simulink model "ofdmexample1"  (R2017a)
settings: Solver=FixedStepDiscrete  StartTime=0.0  StopTime=0.1  RelTol=1e-3
PostLoadFcn:
  | prm80216d.blkh = []; prm80216d.action = 'init';
  | commwman80216d_init(prm80216d.blkh, prm80216d.action);
  | if isempty(ans), clear ans; end
StartFcn:
  | if isempty(ans), clear ans; end
undefined symbols (not defined in the file): idx, magnitude
libraries: commwman80216d_lib x49, dspsigops x24, commcnvcod2 x14, dspindex x4, commdigbbndpm3 x3, dspsolvers x2, simulink x2, commrflib2 x2, commofdm x2, commsink2 x1, commblksprivate x1, dspmtrx3 x1
(part 2 of 2)

== system ofdmexample1/FEC & Modulator Bank/RateID5 - 64 QAM 2//3 ==
  In1 : Inport
  Enable : EnablePort  PropagateVarSize=During execution
  64-QAM Modulator5 : commwman80216d_lib/64-QAM Modulator  SystemSampleTime=-1
      settings: SourceProductName=Communications System Toolbox  SourceProductBaseCode=CM
  Interleaver5 : commwman80216d_lib/Interleaver  numSubCh=16  Ncbps1=1152  Ncbps2=96  Ncbps3=48  Ncbps4=96  Ncbps5=12  Ncpc=6  numSym=prm80216d.numOFDMSymbols
      settings: SourceProductName=Communications System Toolbox  SourceProductBaseCode=CM
  Punctured Convolutional Encoder5 : commcnvcod2/Convolutional Encoder  trellis=poly2trellis(7, [171 133])  opMode=Truncated (reset every frame)  DelayedResetAction=off  hasIniStPort=off  hasFinStPort=off  usePuncVector=on  punctureVector=reshape([1 0 1;1 1 0 ],6,1)  reset=Unused parameter value
      settings: SourceProductName=Communications System Toolbox  SourceProductBaseCode=CM
  RS Encoder5 : commwman80216d_lib/RS Encoder  N=108  K=96  numSym=prm80216d.numOFDMSymbols
      settings: SourceProductName=Communications System Toolbox  SourceProductBaseCode=CM
  Select Bits : dspsigops/Pad  padAlong=Columns  dimsToPad=1  valSrc=Specify via dialog  padVal=0  spec=Output size  padNumOutRowsSpecMethod=User-specified  numOutRows=prm80216d.uncBlkSize(6)*8*prm80216d.numOFDMSymbols - 8  padNumOutColsSpecMethod=User-specified  numOutCols=1  isVarDimsMode=off  padBeginning=0  padEnd=0  outSizeMode=User-specified  outSize=1  padSigAt=End  trunc_flag=None  roundingMode=Floor  overflowMode=off  truncOrWrapMode=Truncate  wrap_flag=None
      settings: AttributesFormatString=\n  SourceProductName=DSP System Toolbox  SourceProductBaseCode=DS
  Zero pad tail byte : dspsigops/Pad  padAlong=Columns  dimsToPad=1  valSrc=Specify via dialog  padVal=0  spec=Output size  padNumOutRowsSpecMethod=User-specified  numOutRows=prm80216d.uncBlkSize(6)*8*prm80216d.numOFDMSymbols  padNumOutColsSpecMethod=User-specified  numOutCols=1  isVarDimsMode=off  padBeginning=0  padEnd=0  outSizeMode=User-specified  outSize=1  padSigAt=End  trunc_flag=None  roundingMode=Floor  overflowMode=off  truncOrWrapMode=Truncate  wrap_flag=None
      settings: AttributesFormatString=\n  SourceProductName=DSP System Toolbox  SourceProductBaseCode=DS
  Out1 : Outport
  wires:
  RS Encoder5/1 -> Punctured Convolutional Encoder5/1
  Punctured Convolutional Encoder5/1 -> Interleaver5/1
  Interleaver5/1 -> 64-QAM Modulator5/1
  In1/1 -> Select Bits/1
  64-QAM Modulator5/1 -> Out1/1
  Select Bits/1 -> Zero pad tail byte/1
  Zero pad tail byte/1 -> RS Encoder5/1

== system ofdmexample1/FEC & Modulator Bank/RateID6 - 64QAM 3//4 ==
  In1 : Inport
  Enable : EnablePort  PropagateVarSize=During execution
  64-QAM Modulator6 : commwman80216d_lib/64-QAM Modulator  SystemSampleTime=-1
      settings: SourceProductName=Communications System Toolbox  SourceProductBaseCode=CM
  Interleaver6 : commwman80216d_lib/Interleaver  numSubCh=16  Ncbps1=1152  Ncbps2=96  Ncbps3=48  Ncbps4=96  Ncbps5=12  Ncpc=6  numSym=prm80216d.numOFDMSymbols
      settings: SourceProductName=Communications System Toolbox  SourceProductBaseCode=CM
  Punctured Convolutional Encoder6 : commcnvcod2/Convolutional Encoder  trellis=poly2trellis(7, [171 133])  opMode=Truncated (reset every frame)  DelayedResetAction=off  hasIniStPort=off  hasFinStPort=off  usePuncVector=on  punctureVector=reshape([1 0 1 0 1;1 1 0 1 0], 10, 1)  reset=Unused parameter value
      settings: SourceProductName=Communications System Toolbox  SourceProductBaseCode=CM
  RS Encoder6 : commwman80216d_lib/RS Encoder  N=120  K=108  numSym=prm80216d.numOFDMSymbols
      settings: SourceProductName=Communications System Toolbox  SourceProductBaseCode=CM
  Select Bits : dspsigops/Pad  padAlong=Columns  dimsToPad=1  valSrc=Specify via dialog  padVal=0  spec=Output size  padNumOutRowsSpecMethod=User-specified  numOutRows=prm80216d.uncBlkSize(7)*8*prm80216d.numOFDMSymbols - 8  padNumOutColsSpecMethod=User-specified  numOutCols=1  isVarDimsMode=off  padBeginning=0  padEnd=0  outSizeMode=User-specified  outSize=1  padSigAt=End  trunc_flag=None  roundingMode=Floor  overflowMode=off  truncOrWrapMode=Truncate  wrap_flag=None
      settings: AttributesFormatString=\n  SourceProductName=DSP System Toolbox  SourceProductBaseCode=DS
  Zero pad tail byte : dspsigops/Pad  padAlong=Columns  dimsToPad=1  valSrc=Specify via dialog  padVal=0  spec=Output size  padNumOutRowsSpecMethod=User-specified  numOutRows=prm80216d.uncBlkSize(7)*8*prm80216d.numOFDMSymbols  padNumOutColsSpecMethod=User-specified  numOutCols=1  isVarDimsMode=off  padBeginning=0  padEnd=0  outSizeMode=User-specified  outSize=1  padSigAt=End  trunc_flag=None  roundingMode=Floor  overflowMode=off  truncOrWrapMode=Truncate  wrap_flag=None
      settings: AttributesFormatString=\n  SourceProductName=DSP System Toolbox  SourceProductBaseCode=DS
  Out1 : Outport
  wires:
  RS Encoder6/1 -> Punctured Convolutional Encoder6/1
  Punctured Convolutional Encoder6/1 -> Interleaver6/1
  Interleaver6/1 -> 64-QAM Modulator6/1
  In1/1 -> Select Bits/1
  64-QAM Modulator6/1 -> Out1/1
  Select Bits/1 -> Zero pad tail byte/1
  Zero pad tail byte/1 -> RS Encoder6/1

== system ofdmexample1/Subsystem2/Subsystem1 ==
  Modulated Preamble : Constant  Value=prm80216d.modedPreamble  VectorParams1D=off
  Out : Outport
  wires:
  Modulated Preamble/1 -> Out/1

== system ofdmexample1/Compensator/Compensator/Gains ==
  ch est : Inport
  Math Function : Math  Operator=magnitude^2  SaturateOnIntegerOverflow=on
  Math Function1 : Math  Operator=conj  SaturateOnIntegerOverflow=on
  Product3 : Product  Inputs=*/  SaturateOnIntegerOverflow=on  OutDataTypeStr=Inherit: Same as first input
  Repeat : dspsigops/Repeat  N=prm80216d.numOFDMSymbols  InputProcessing=Columns as channels (frame based)  RateOptions=Enforce single-rate processing  ic=0  mode=Unused parameter value
      settings: SourceProductName=DSP System Toolbox
  Transpose : Math  Operator=transpose  SaturateOnIntegerOverflow=on
  Transpose1 : Math  Operator=transpose  SaturateOnIntegerOverflow=on
  gains : Outport
  wires:
  Product3/1 -> Repeat/1
  Transpose1/1 -> gains/1
  Repeat/1 -> Transpose1/1
  Transpose/1 -> Math Function/1, Math Function1/1
  Math Function1/1 -> Product3/1
  Math Function/1 -> Product3/2
  ch est/1 -> Transpose/1

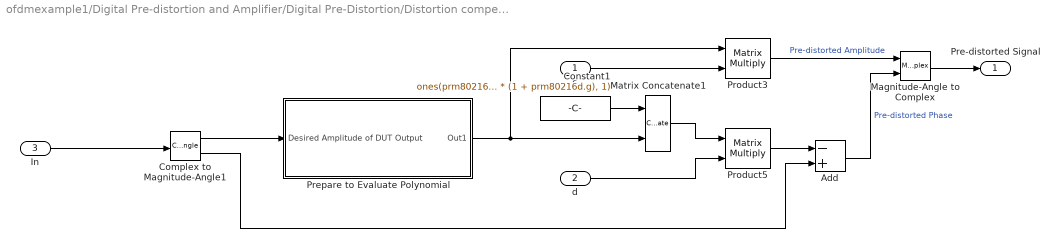
== system ofdmexample1/Digital Pre-distortion and Amplifier/Digital Pre-Distortion/Distortion compensation ==
  c : Inport
  d : Inport  Port=2
  In : Inport  Port=3
  Add : Sum  Inputs=-+
  Complex to Magnitude-Angle1 : ComplexToMagnitudeAngle
  Constant1 : Constant  Value=ones(prm80216d.totOFDMSym * prm80216d.nfft * (1 + prm80216d.g), 1)
  Magnitude-Angle to Complex : MagnitudeAngleToComplex
  Matrix Concatenate1 : Concatenate  Mode=Multidimensional array  ConcatenateDimension=2
  Prepare to Evaluate Polynomial : Subsystem
  Product3 : Product  Multiplication=Matrix(*)  RndMeth=Zero
  Product5 : Product  Multiplication=Matrix(*)  RndMeth=Zero
  Pre-distorted Signal : Outport
  wires:
  c/1 -> Product3/2
  Add/1 -> Magnitude-Angle to Complex/2  "Pre-distorted Phase"
  Product5/1 -> Add/1
  Product3/1 -> Magnitude-Angle to Complex/1  "Pre-distorted Amplitude"
  d/1 -> Product5/2
  In/1 -> Complex to Magnitude-Angle1/1
  Magnitude-Angle to Complex/1 -> Pre-distorted Signal/1
  Complex to Magnitude-Angle1/2 -> Add/2
  Complex to Magnitude-Angle1/1 -> Prepare to Evaluate Polynomial/1(Desired Amplitude of DUT Output)
  Matrix Concatenate1/1 -> Product5/1
  Prepare to Evaluate Polynomial/1(Out1) -> Matrix Concatenate1/2, Product3/1
  Constant1/1 -> Matrix Concatenate1/1

== system ofdmexample1/Digital Pre-distortion and Amplifier/Digital Pre-Distortion/Parameter Estimation ==
  DUT Input : Inport
  DUT Output : Inport  Port=2
  Complex to Magnitude-Angle : ComplexToMagnitudeAngle
  Complex to Magnitude-Angle1 : ComplexToMagnitudeAngle
  Polynomial Approximation : Subsystem
  c : Outport
  d : Outport  Port=2
  wires:
  DUT Input/1 -> Complex to Magnitude-Angle/1
  DUT Output/1 -> Complex to Magnitude-Angle1/1
  Complex to Magnitude-Angle1/1 -> Polynomial Approximation/3(Amplitude of DUT Output)
  Complex to Magnitude-Angle/2 -> Polynomial Approximation/2(Phase of DUT Input)
  Polynomial Approximation/1(Coef_c) -> c/1
  Polynomial Approximation/2(Coef_d) -> d/1
  Complex to Magnitude-Angle1/2 -> Polynomial Approximation/4(Phase of DUT Output)
  Complex to Magnitude-Angle/1 -> Polynomial Approximation/1(Amplitude of DUT Input)

== system ofdmexample1/Digital Pre-distortion and Amplifier/Digital Pre-Distortion/Distortion compensation/Prepare to Evaluate Polynomial ==
  Desired Amplitude of DUT Output : Inport
  Matrix Concatenate1 : Concatenate  NumInputs=5  Mode=Multidimensional array  ConcatenateDimension=2
  Product{6..9} (4 alike) : Product  RndMeth=Zero
  Out1 : Outport
  wires:
  Desired Amplitude of DUT Output/1 -> Product9/2, Product8/2, Product7/2, Product6/2, Product6/1, Matrix Concatenate1/1
  Product7/1 -> Product8/1, Matrix Concatenate1/3
  Product6/1 -> Product7/1, Matrix Concatenate1/2
  Product8/1 -> Product9/1, Matrix Concatenate1/4
  Product9/1 -> Matrix Concatenate1/5
  Matrix Concatenate1/1 -> Out1/1

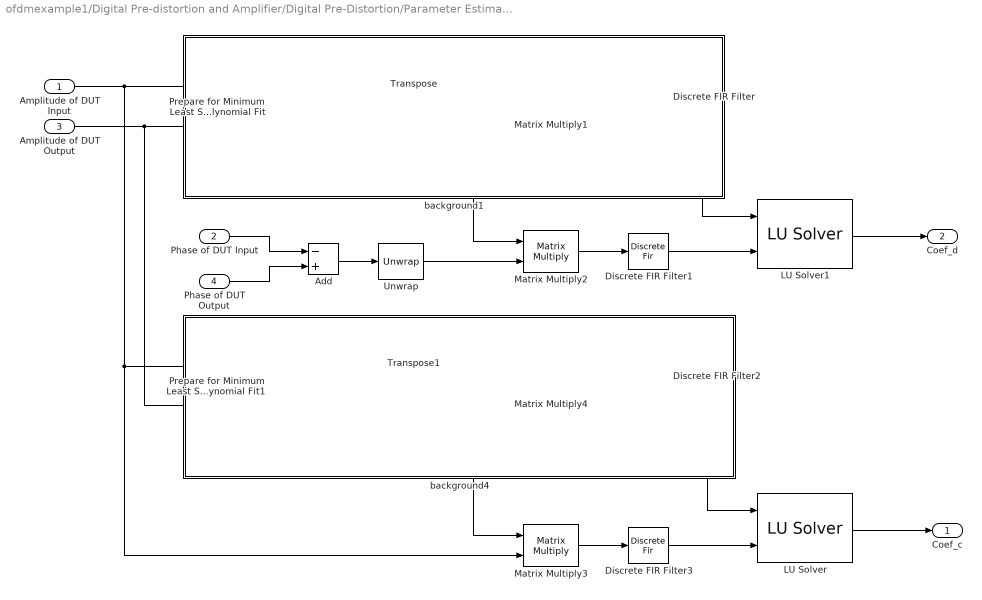
== system ofdmexample1/Digital Pre-distortion and Amplifier/Digital Pre-Distortion/Parameter Estimation/Polynomial Approximation ==
  Amplitude of DUT Input : Inport
  Phase of DUT Input : Inport  Port=2
  Amplitude of DUT Output : Inport  Port=3
  Phase of DUT Output : Inport  Port=4
  Add : Sum  Inputs=-+
  Discrete FIR Filter{,1..3} (4 alike) : DiscreteFir  Coefficients=ones(1,50)  AccumDataTypeStr=Inherit: Same as product output
  LU Solver : dspsolvers/LU Solver
      settings: SourceProductName=DSP System Toolbox  SourceProductBaseCode=DS
  LU Solver1 : dspsolvers/LU Solver
      settings: SourceProductName=DSP System Toolbox  SourceProductBaseCode=DS
  Matrix Multiply{1..4} (4 alike) : Product  Multiplication=Matrix(*)
  Prepare for Minimum Least Square Error Polynomial Fit : Subsystem
  Prepare for Minimum Least Square Error Polynomial Fit1 : Subsystem
  Transpose : Math  Operator=transpose  SaturateOnIntegerOverflow=on
  Transpose1 : Math  Operator=transpose  SaturateOnIntegerOverflow=on
  Unwrap : dspsigops/Unwrap  tol=pi  InputProcessing=Columns as channels (frame based)  running=off
  background1 : Subsystem
      mask Display: disp('')
  background4 : Subsystem
      mask Display: disp('')
  Coef_c : Outport
  Coef_d : Outport  Port=2
  wires:
  Discrete FIR Filter2/1 -> LU Solver/1
  Transpose1/1 -> Matrix Multiply3/1, Matrix Multiply4/1
  Matrix Multiply4/1 -> Discrete FIR Filter2/1
  Prepare for Minimum Least Square Error Polynomial Fit1/1(Out1) -> Matrix Multiply4/2, Transpose1/1
  Phase of DUT Input/1 -> Add/1
  Add/1 -> Unwrap/1
  Amplitude of DUT Input/1 -> Prepare for Minimum Least Square Error Polynomial Fit/1(In1), Prepare for Minimum Least Square Error Polynomial Fit1/1(In1), Matrix Multiply3/2
  Matrix Multiply1/1 -> Discrete FIR Filter/1
  Matrix Multiply3/1 -> Discrete FIR Filter3/1
  Prepare for Minimum Least Square Error Polynomial Fit/1(Out1) -> Matrix Multiply1/2, Transpose/1
  Unwrap/1 -> Matrix Multiply2/2
  Matrix Multiply2/1 -> Discrete FIR Filter1/1
  Amplitude of DUT Output/1 -> Prepare for Minimum Least Square Error Polynomial Fit1/2(In2), Prepare for Minimum Least Square Error Polynomial Fit/2(In2)
  Discrete FIR Filter1/1 -> LU Solver1/2
  Discrete FIR Filter/1 -> LU Solver1/1
  Discrete FIR Filter3/1 -> LU Solver/2
  Phase of DUT Output/1 -> Add/2
  LU Solver1/1 -> Coef_d/1
  LU Solver/1 -> Coef_c/1
  Transpose/1 -> Matrix Multiply1/1, Matrix Multiply2/1

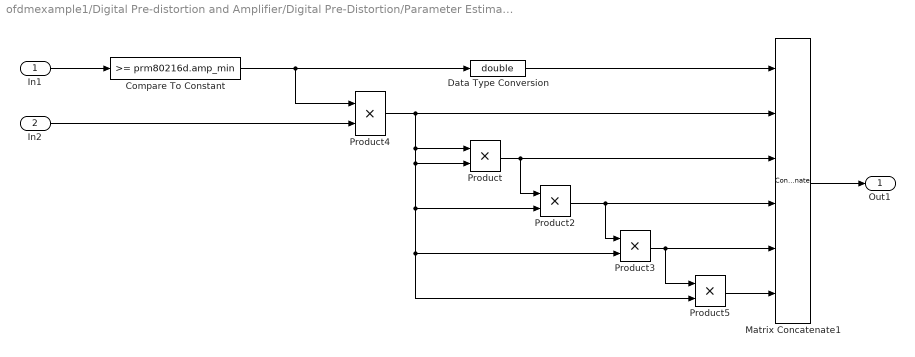
== system ofdmexample1/Digital Pre-distortion and Amplifier/Digital Pre-Distortion/Parameter Estimation/Polynomial Approximation/Prepare for Minimum Least Square Error Polynomial Fit ==
  In1 : Inport
  In2 : Inport  Port=2
  Compare To Constant : simulink/Logic and Bit Operations/Compare To Constant  relop=>=  const=prm80216d.amp_min  OutDataTypeStr=uint8  ZeroCross=off
  Data Type Conversion : DataTypeConversion  OutDataTypeStr=double
  Matrix Concatenate1 : Concatenate  NumInputs=6  Mode=Multidimensional array  ConcatenateDimension=2
  Product{,2..5} (5 alike) : Product  RndMeth=Zero
  Out1 : Outport
  wires:
  Compare To Constant/1 -> Product4/1, Data Type Conversion/1
  In2/1 -> Product4/2
  Product3/1 -> Product5/1, Matrix Concatenate1/5
  Product2/1 -> Product3/1, Matrix Concatenate1/4
  Product/1 -> Product2/1, Matrix Concatenate1/3
  Product4/1 -> Product5/2, Product3/2, Product2/2, Product/2, Product/1, Matrix Concatenate1/2
  Product5/1 -> Matrix Concatenate1/6
  Matrix Concatenate1/1 -> Out1/1
  In1/1 -> Compare To Constant/1
  Data Type Conversion/1 -> Matrix Concatenate1/1

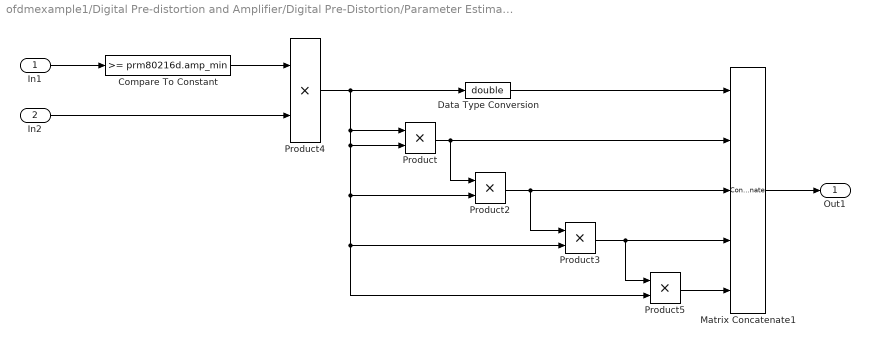
== system ofdmexample1/Digital Pre-distortion and Amplifier/Digital Pre-Distortion/Parameter Estimation/Polynomial Approximation/Prepare for Minimum Least Square Error Polynomial Fit1 ==
  In1 : Inport
  In2 : Inport  Port=2
  Compare To Constant : simulink/Logic and Bit Operations/Compare To Constant  relop=>=  const=prm80216d.amp_min  OutDataTypeStr=uint8  ZeroCross=off
  Data Type Conversion : DataTypeConversion  OutDataTypeStr=double
  Matrix Concatenate1 : Concatenate  NumInputs=5  Mode=Multidimensional array  ConcatenateDimension=2
  Product{,2..5} (5 alike) : Product  RndMeth=Zero
  Out1 : Outport
  wires:
  Compare To Constant/1 -> Product4/1
  Data Type Conversion/1 -> Matrix Concatenate1/1
  In2/1 -> Product4/2
  Product/1 -> Product2/1, Matrix Concatenate1/2
  Product4/1 -> Data Type Conversion/1, Product3/2, Product5/2, Product2/2, Product/2, Product/1
  Product5/1 -> Matrix Concatenate1/5
  Product3/1 -> Matrix Concatenate1/4, Product5/1
  Product2/1 -> Matrix Concatenate1/3, Product3/1
  Matrix Concatenate1/1 -> Out1/1
  In1/1 -> Compare To Constant/1

== system ofdmexample1/Digital Pre-distortion and Amplifier/Digital Pre-Distortion/Parameter Estimation/Polynomial Approximation/background1 ==

== system ofdmexample1/Digital Pre-distortion and Amplifier/Digital Pre-Distortion/Parameter Estimation/Polynomial Approximation/background4 ==
